simulink subsystem "FOC_Sub_CoreAlgoithm"  (R2025b)
settings: Solver=VariableStepAuto  StartTime=0.0  StopTime=10.0  RelTol=1e-3
PreLoadFcn:
  | FOC_Config;
undefined symbols (not defined in the file): innerPI, motor, outerPI, Tctr
libraries: mcbeeMathTransformLib x3, slpidlib x3, mcbcontrolslib x3, mcbpositiondecoderlib x2
settings Model: Creator=k  LastModifiedBy=k
settings SolverCC: AlgebraicLoopSolver=TrustRegion
settings DebuggingCC: UnconnectedInputMsg=warning  UnconnectedOutputMsg=warning  UnconnectedLineMsg=warning
settings ModelReferenceCC: EnableRefExpFcnMdlSchedulingChecks=on
settings RTWCC: GPUComputeCapability=3.5  DLArmComputeVersion=19.05

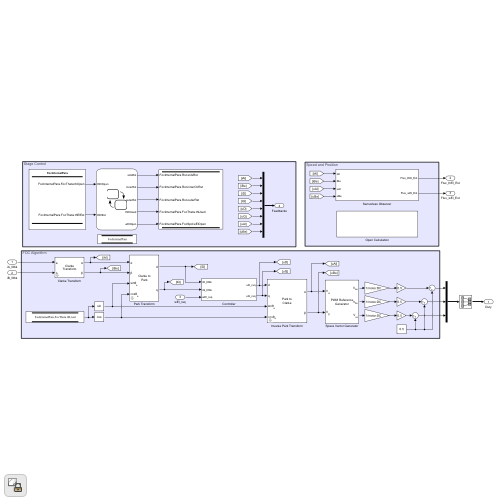
[thumbnail: Simulink's stored preview of the top-level diagram]
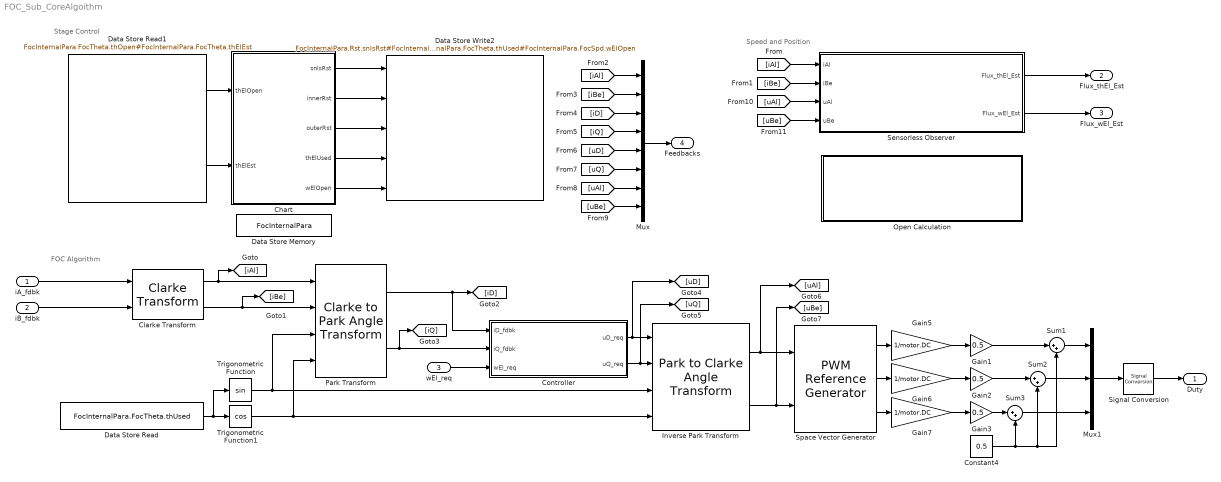
== system FOC_Sub_CoreAlgoithm ==
  note: Speed and Position
  note: Stage Control
  note: FOC Algorithm
  iA_fdbk : Inport
  iB_fdbk : Inport  Port=2
  wEl_req : Inport  Port=3
  Chart : Stateflow chart  TreatAsAtomicUnit=on
  Clarke Transform : mcbeeMathTransformLib/Clarke Transform  VariantControl=Variant2  PowerInvariant=off  UseWithEmbedded=on  PhaseInput=Two inputs
  Constant4 : Constant  Value=0.5  OutDataTypeStr=single
  Controller : Subsystem
  Data Store Memory : DataStoreMemory  DataStoreName=FocInternalPara  ReadBeforeWriteMsg=warning  WriteAfterWriteMsg=warning  WriteAfterReadMsg=warning  ShowAdditionalParam=off  OutDataTypeStr=Bus: strcutFocInternalPara
  Data Store Read : DataStoreRead  DataStoreName=FocInternalPara  DataStoreElements=FocInternalPara.FocTheta.thUsed  IndexOptions=Index vector (dialog)  Indices=1  OutputSizes=1
  Data Store Read1 : DataStoreRead  DataStoreName=FocInternalPara  DataStoreElements=FocInternalPara.FocTheta.thOpen#FocInternalPara.FocTheta.thElEst  IndexOptions=Index vector (dialog)  Indices=1  OutputSizes=1
  Data Store Write2 : DataStoreWrite  DataStoreName=FocInternalPara  DataStoreElements=FocInternalPara.Rst.snlsRst#FocInternalPara.Rst.innerCtrRst#FocInternalPara.Rst.outerRst#FocInternalPara.FocTheta.thUsed#FocInternalPara.FocSpd.wElOpen  IndexOptions=Index vector (dialog)  Indices=1  OutputSizes=1
  Gain1 : Gain  Gain=0.5  OutDataTypeStr=single
  Gain2 : Gain  Gain=0.5  OutDataTypeStr=single
  Gain3 : Gain  Gain=0.5  OutDataTypeStr=single
  Gain5 : Gain  Gain=1/motor.DC
  Gain6 : Gain  Gain=1/motor.DC
  Gain7 : Gain  Gain=1/motor.DC
  Inverse Park Transform : mcbeeMathTransformLib/Park to Clarke Angle Transform  AxisAlignment=D-axis  UseWithEmbedded=on  PhaseInput=Two inputs  ThetaInput=Sine and Cosine electrical position  AngleInput=Per-unit  N_points=1024
  Mux : Mux  Inputs=8
  Mux1 : Mux  Inputs=3
  Open Calculation : Subsystem
  Park Transform : mcbeeMathTransformLib/Clarke to Park Angle Transform  AxisAlignment=D-axis  UseWithEmbedded=on  PhaseInput=Two inputs  ThetaInput=Sine and Cosine electrical position  AngleInput=Per-unit  N_points=1024
  Sensorless Observer : Subsystem
  Signal Conversion : SignalConversion  OverrideOpt=off
  Space Vector Generator : mcbcontrolslib/PWM Reference Generator  inSignal=Valphabeta  modType=SVM: space vector modulation
  Sum1 : Sum  Inputs=|++
  Sum2 : Sum  Inputs=|++
  Sum3 : Sum  Inputs=|++
  Trigonometric Function : Trigonometry
  Trigonometric Function1 : Trigonometry  Operator=cos
  Duty : Outport  PortDimensions=3
  Flux_thEl_Est : Outport  Port=2
  Flux_wEl_Est : Outport  Port=3
  Feedbacks : Outport  Port=4
  wires:
  Signal Conversion/1 -> Duty/1
  Mux1/1 -> Signal Conversion/1
  Sum1/1 -> Mux1/1
  Sum3/1 -> Mux1/3
  Sum2/1 -> Mux1/2
  iB_fdbk/1 -> Clarke Transform/2
  iA_fdbk/1 -> Clarke Transform/1
  Clarke Transform/1 -> Park Transform/1, [iAl]
  Clarke Transform/2 -> [iBe], Park Transform/2
  Gain7/1 -> Gain3/1
  Constant4/1 -> Sum3/2, Sum2/2, Sum1/2
  Space Vector Generator/1 -> Gain5/1
  Space Vector Generator/2 -> Gain6/1
  Gain5/1 -> Gain1/1
  Gain1/1 -> Sum1/1
  Space Vector Generator/3 -> Gain7/1
  Gain2/1 -> Sum2/1
  Gain3/1 -> Sum3/1
  Gain6/1 -> Gain2/1
  Inverse Park Transform/1 -> Space Vector Generator/1, [uAl]
  Inverse Park Transform/2 -> [uBe], Space Vector Generator/2
  Sensorless Observer/1(Flux_thEl_Est) -> Flux_thEl_Est/1
  Sensorless Observer/2(Flux_wEl_Est) -> Flux_wEl_Est/1
  Park Transform/1 -> Controller/1(iD_fdbk), [iD]
  Park Transform/2 -> [iQ], Controller/2(iQ_fdbk)
  Controller/1(uD_req) -> Inverse Park Transform/1, [uD]
  Controller/2(uQ_req) -> [uQ], Inverse Park Transform/2
  Trigonometric Function1/1 -> Park Transform/4, Inverse Park Transform/4
  Data Store Read/1 -> Trigonometric Function/1, Trigonometric Function1/1
  Trigonometric Function/1 -> Park Transform/3, Inverse Park Transform/3
  wEl_req/1 -> Controller/3(wEl_req)
  Chart/3(outerRst) -> Data Store Write2/3
  Chart/2(innerRst) -> Data Store Write2/2
  Chart/1(snlsRst) -> Data Store Write2/1
  Data Store Read1/1 -> Chart/1(thElOpen)
  Data Store Read1/2 -> Chart/2(thElEst)
  Chart/4(thElUsed) -> Data Store Write2/4
  Chart/5(wElOpen) -> Data Store Write2/5
  [iAl] -> Sensorless Observer/1(iAl)
  [iBe] -> Sensorless Observer/2(iBe)
  [uAl] -> Sensorless Observer/3(uAl)
  [uBe] -> Sensorless Observer/4(uBe)
  [uBe] -> Mux/8
  [uAl] -> Mux/7
  [uQ] -> Mux/6
  [uD] -> Mux/5
  [iQ] -> Mux/4
  [iD] -> Mux/3
  [iBe] -> Mux/2
  [iAl] -> Mux/1
  Mux/1 -> Feedbacks/1

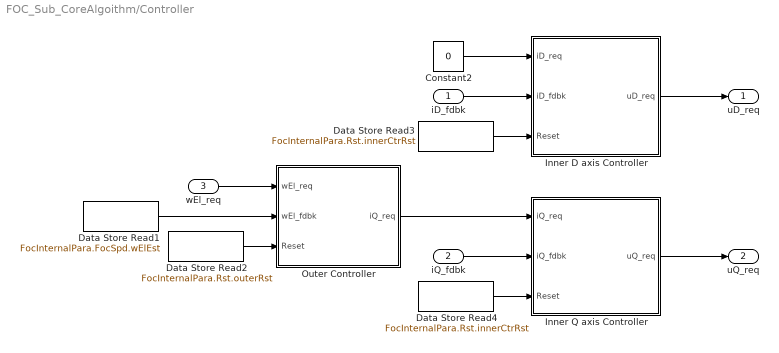
== system FOC_Sub_CoreAlgoithm/Controller ==
  iD_fdbk : Inport
  iQ_fdbk : Inport  Port=2
  wEl_req : Inport  Port=3
  Constant2 : Constant  Value=0  OutDataTypeStr=single
  Data Store Read1 : DataStoreRead  DataStoreName=FocInternalPara  DataStoreElements=FocInternalPara.FocSpd.wElEst  IndexOptions=Index vector (dialog)  Indices=1  OutputSizes=1
  Data Store Read2 : DataStoreRead  DataStoreName=FocInternalPara  DataStoreElements=FocInternalPara.Rst.outerRst  IndexOptions=Index vector (dialog)  Indices=1  OutputSizes=1
  Data Store Read3 : DataStoreRead  DataStoreName=FocInternalPara  DataStoreElements=FocInternalPara.Rst.innerCtrRst  IndexOptions=Index vector (dialog)  Indices=1  OutputSizes=1
  Data Store Read4 : DataStoreRead  DataStoreName=FocInternalPara  DataStoreElements=FocInternalPara.Rst.innerCtrRst  IndexOptions=Index vector (dialog)  Indices=1  OutputSizes=1
  Inner D axis Controller : Subsystem
  Inner Q axis Controller : Subsystem
  Outer Controller : Subsystem
  uD_req : Outport
  uQ_req : Outport  Port=2
  wires:
  Inner D axis Controller/1(uD_req) -> uD_req/1
  iD_fdbk/1 -> Inner D axis Controller/2(iD_fdbk)
  wEl_req/1 -> Outer Controller/1(wEl_req)
  Data Store Read1/1 -> Outer Controller/2(wEl_fdbk)
  Constant2/1 -> Inner D axis Controller/1(iD_req)
  Inner Q axis Controller/1(uQ_req) -> uQ_req/1
  Data Store Read2/1 -> Outer Controller/3(Reset)
  Outer Controller/1(iQ_req) -> Inner Q axis Controller/1(iQ_req)
  iQ_fdbk/1 -> Inner Q axis Controller/2(iQ_fdbk)
  Data Store Read3/1 -> Inner D axis Controller/3(Reset)
  Data Store Read4/1 -> Inner Q axis Controller/3(Reset)

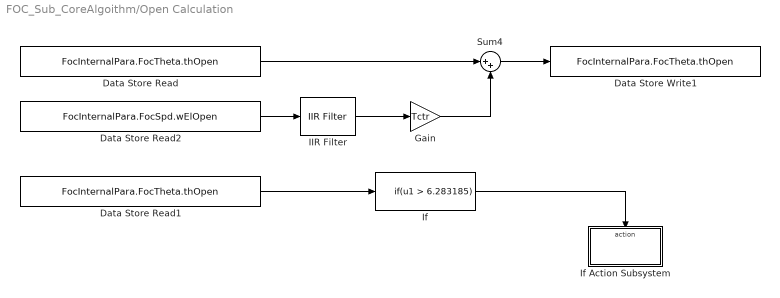
== system FOC_Sub_CoreAlgoithm/Open Calculation ==
  Data Store Read : DataStoreRead  DataStoreName=FocInternalPara  DataStoreElements=FocInternalPara.FocTheta.thOpen  IndexOptions=Index vector (dialog)  Indices=1  OutputSizes=1
  Data Store Read1 : DataStoreRead  DataStoreName=FocInternalPara  DataStoreElements=FocInternalPara.FocTheta.thOpen  IndexOptions=Index vector (dialog)  Indices=1  OutputSizes=1
  Data Store Read2 : DataStoreRead  DataStoreName=FocInternalPara  DataStoreElements=FocInternalPara.FocSpd.wElOpen  IndexOptions=Index vector (dialog)  Indices=1  OutputSizes=1
  Data Store Write1 : DataStoreWrite  DataStoreName=FocInternalPara  DataStoreElements=FocInternalPara.FocTheta.thOpen  IndexOptions=Index vector (dialog)  Indices=1  OutputSizes=1
  Gain : Gain  Gain=Tctr
  IIR Filter : mcbcontrolslib/IIR Filter  VariantControl=Low Pass Filter  VariantSelect=Low-pass  FilterConstantInputType=Specify via dialog  Filter_constant=0.002  InitialOutput=Specify via dialog  InitialOutputValue=0  ExternalReset=none  advancedSettings=off  Ts=50e-6  cutOff_freq=6.379
  If : If  IfExpression=u1 > 6.283185  ShowElse=off
  If Action Subsystem : Subsystem  TreatAsAtomicUnit=on
  Sum4 : Sum  Inputs=|++  OutDataTypeStr=single
  wires:
  If/1 -> If Action Subsystem/Action
  Data Store Read1/1 -> If/1
  Data Store Read/1 -> Sum4/1
  Sum4/1 -> Data Store Write1/1
  Data Store Read2/1 -> IIR Filter/1
  Gain/1 -> Sum4/2
  IIR Filter/1 -> Gain/1

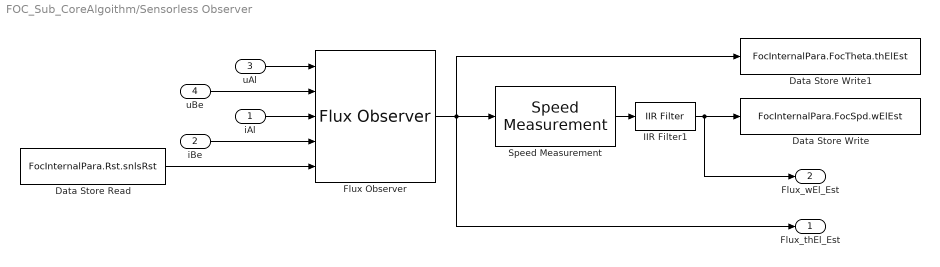
== system FOC_Sub_CoreAlgoithm/Sensorless Observer ==
  iAl : Inport
  iBe : Inport  Port=2
  uAl : Inport  Port=3
  uBe : Inport  Port=4
  Data Store Read : DataStoreRead  DataStoreName=FocInternalPara  DataStoreElements=FocInternalPara.Rst.snlsRst  IndexOptions=Index vector (dialog)  Indices=1  OutputSizes=1
  Data Store Write : DataStoreWrite  DataStoreName=FocInternalPara  DataStoreElements=FocInternalPara.FocSpd.wElEst  IndexOptions=Index vector (dialog)  Indices=1  OutputSizes=1
  Data Store Write1 : DataStoreWrite  DataStoreName=FocInternalPara  DataStoreElements=FocInternalPara.FocTheta.thElEst  IndexOptions=Index vector (dialog)  Indices=1  OutputSizes=1
  Flux Observer : mcbpositiondecoderlib/Flux Observer  DataTypeSelect=off  ParameterBusInput=off  MotorSelection=PMSM  BlockInputUnit=SI unit  PerUnitVoltage=13.86  PerUnitCurrent=19.3  PositionSelect=on  FluxSelect=off  TorqueSelect=off  PolePairs=4  StatorResistance=motor.Rs  StatorDAxisInductance=motor.L0*2  StatorLeakageInductance=0.0068  RotorLeakageInductance=0.0068  MagnetizingInductance=0.0300  CutoffFreq=3.1863  BlockSampleTime=Tctr  PositionUnit=Radians  PositionDatatype=single  FluxUnit=Weber  PerUnitFlux=0.1  FluxDatatype=single  TorqueUnit=Nm  PerUnitTorque=100  TorqueDatatype=single  DataType=0
  IIR Filter1 : mcbcontrolslib/IIR Filter  VariantControl=Low Pass Filter  VariantSelect=Low-pass  FilterConstantInputType=Specify via dialog  Filter_constant=0.001  InitialOutput=Specify via dialog  InitialOutputValue=0  ExternalReset=none  advancedSettings=off  Ts=50e-6  cutOff_freq=3.1863
  Speed Measurement : mcbpositiondecoderlib/Speed Measurement  DiscreteStepInput=off  LastDiscreteStepInput=off  PositionUnit=Radians  PositionScalingDatatype=uint32  SpeedCalculationMode=Time interval for speed calculation  TempSpeedCalculationMode=Time interval for speed calculation  SampleTimeAsync=Tctr  MaximumApplicationSpeed=1000  SpeedResolution=5e-6  DelayLength=20  MaximumMeasurableSpeed=22857.1429  MeasurableSpeedResolution=1.1176e-05  SpeedUnit=Radians/Sec  TempSpeedUnit=RPM  PerUnitSpeed=1000  SpeedDataType=single
  Flux_thEl_Est : Outport
  Flux_wEl_Est : Outport  Port=2
  wires:
  iBe/1 -> Flux Observer/4
  uBe/1 -> Flux Observer/2
  IIR Filter1/1 -> Data Store Write/1, Flux_wEl_Est/1
  Speed Measurement/1 -> IIR Filter1/1
  uAl/1 -> Flux Observer/1
  iAl/1 -> Flux Observer/3
  Data Store Read/1 -> Flux Observer/5
  Flux Observer/1 -> Speed Measurement/1, Flux_thEl_Est/1, Data Store Write1/1

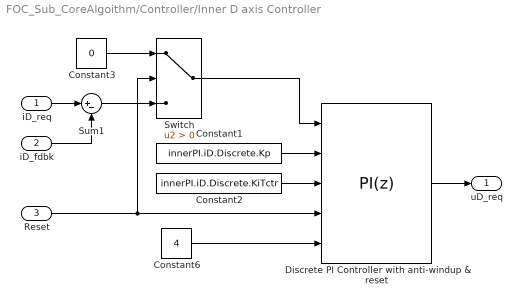
== system FOC_Sub_CoreAlgoithm/Controller/Inner D axis Controller ==
  iD_req : Inport
  iD_fdbk : Inport  Port=2
  Reset : Inport  Port=3
  Constant1 : Constant  Value=innerPI.iD.Discrete.Kp  OutDataTypeStr=single
  Constant2 : Constant  Value=innerPI.iD.Discrete.KiTctr  OutDataTypeStr=single
  Constant3 : Constant  Value=0  OutDataTypeStr=single
  Constant6 : Constant  Value=4  OutDataTypeStr=single
  Discrete PI Controller with anti-windup & reset : slpidlib/PID Controller  Controller=PI  Form=Parallel  TimeDomain=Discrete-time  UseExternalTs=off  SampleTime=-1  IntegratorMethod=Forward Euler  FilterMethod=Forward Euler  ControllerParametersSource=external  P=1  I=1  UseKiTs=on  D=0  UseExternalDerivativeSource=off  N=100  UseFilter=on  TunerSelectOption=Transfer Function Based (PID Tuner App)  InitialConditionSource=external  InitialConditionForIntegrator=0  InitialConditionForFilter=0  DifferentiatorICPrevScaledInput=0  ExternalReset=level  TrackingMode=off  Kt=1  LimitOutput=on  SatLimitsSource=internal  UpperSaturationLimit=10  LowerSaturationLimit=-10  LinearizeAsGain=on  AntiWindupMode=clamping  Kb=1  LimitIntegrator=off  UpperIntegratorSaturationLimit=inf  LowerIntegratorSaturationLimit=-inf  RndMeth=Simplest  POutMin=[]  POutMax=[]  IOutMin=[]  IOutMax=[]  DOutMin=[]  DOutMax=[]  NOutMin=[]  NOutMax=[]  SumOutMin=[]  SumOutMax=[]  SaturationOutDataTypeStr=Inherit: Inherit via back propagation  SaturationOutMin=[]  SaturationOutMax=[]  PParamMin=[]  PParamMax=[]  IParamMin=[]  IParamMax=[]  DParamMin=[]  DParamMax=[]  NParamMin=[]  NParamMax=[]  KbParamMin=[]  KbParamMax=[]  KtParamMin=[]  KtParamMax=[]  KbOutMin=[]  KbOutMax=[]  KtOutMin=[]  KtOutMax=[]  IntegratorOutMin=[]  IntegratorOutMax=[]  FilterOutMin=[]  FilterOutMax=[]  SumI1OutMin=[]  SumI1OutMax=[]  SumI2OutMin=[]  SumI2OutMax=[]  SumI3OutMin=[]  SumI3OutMax=[]  SumI4OutMin=[]  SumI4OutMax=[]  SumDOutMin=[]  SumDOutMax=[]  DifferentiatorOutMin=[]  DifferentiatorOutMax=[]  FilterDiffOutCoefMin=[]  FilterDiffOutCoefMax=[]  ReciprocalOutMin=[]  ReciprocalOutMax=[]  SumDenOutMin=[]  SumDenOutMax=[]  SumNumOutMin=[]  SumNumOutMax=[]  DivideOutMin=[]  DivideOutMax=[]  UdiffTsProdOutMin=[]  UdiffTsProdOutMax=[]  NTsProdOutMin=[]  NTsProdOutMax=[]  UintegralTsProdOutMin=[]  UintegralTsProdOutMax=[]  UngainTsProdOutMin=[]  UngainTsProdOutMax=[]  ClampingZeroOutDataTypeStr=Inherit: Inherit via back propagation  ClampingZeroOutMin=[]  ClampingZeroOutMax=[]  FilterDenConstantOutDataTypeStr=Inherit: Inherit via back propagation  FilterDenConstantOutMin=[]  FilterDenConstantOutMax=[]  PCopyOutDataTypeStr=Inherit: Inherit via back propagation  PCopyOutMin=[]  PCopyOutMax=[]  NCopyOutDataTypeStr=Inherit: Inherit via back propagation  NCopyOutMin=[]  NCopyOutMax=[]  IntegratorContinuousStateAttributes=''  IntegratorStateMustResolveToSignalObject=off  IntegratorRTWStateStorageClass=Auto  FilterContinuousStateAttributes=''  FilterStateMustResolveToSignalObject=off  FilterRTWStateStorageClass=Auto  ParallelPVariant=ExternalParameters  IdealPVariant=Disabled  IVariant=ExternalParameters  DVariant=Disabled  IntegratorVariant=Discrete  SatVariant=Enabled  AWVariant=DiscClampingParallel  PCopyVariant=Disabled  TRVariant=Disabled  FdbkBlocksVariant=Forward  IdealPFdbkVariant=Disabled  SatFdbkVariant=Disabled  DerivativeFilterVariant=Disabled  NVariant=Disabled  NCopyVariant=Disabled_SignalSpec  FilterICVariant=Disabled  IntegratorICVariant=ExternalICs  ExternalResetVariant=ExternalReset  TRSumVariant=Passthrough  SumFdbkVariant=Disabled  SumVariant=Sum_PI  TsampFilterVariant=InternalTs  TsampNgainVariant=Passthrough  TsampIntegralVariant=Disabled_SignalSpec  ExternalSaturationOutDataTypeStr=Inherit: Same as second input  DerivativeSourceVariant=Disabled  PreIntVariant=InternalPreInt
  Sum1 : Sum  Inputs=|+-
  Switch : Switch  Criteria=u2 > Threshold  SaturateOnIntegerOverflow=off  InputSameDT=off
  uD_req : Outport
  wires:
  Constant6/1 -> Discrete PI Controller with anti-windup & reset/5
  Discrete PI Controller with anti-windup & reset/1 -> uD_req/1
  Constant2/1 -> Discrete PI Controller with anti-windup & reset/3
  Constant1/1 -> Discrete PI Controller with anti-windup & reset/2
  Reset/1 -> Switch/2, Discrete PI Controller with anti-windup & reset/4
  Constant3/1 -> Switch/1
  iD_fdbk/1 -> Sum1/2
  Sum1/1 -> Switch/3
  iD_req/1 -> Sum1/1
  Switch/1 -> Discrete PI Controller with anti-windup & reset/1

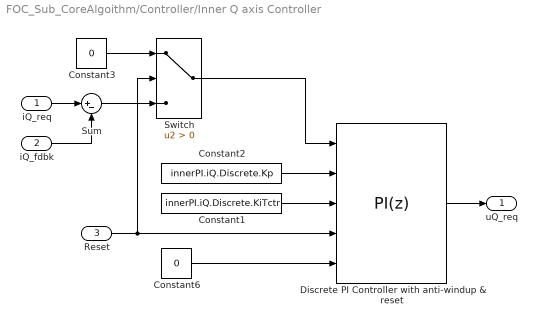
== system FOC_Sub_CoreAlgoithm/Controller/Inner Q axis Controller ==
  iQ_req : Inport
  iQ_fdbk : Inport  Port=2
  Reset : Inport  Port=3
  Constant1 : Constant  Value=innerPI.iQ.Discrete.KiTctr  OutDataTypeStr=single
  Constant2 : Constant  Value=innerPI.iQ.Discrete.Kp  OutDataTypeStr=single
  Constant3 : Constant  Value=0  OutDataTypeStr=single
  Constant6 : Constant  Value=0  OutDataTypeStr=single
  Discrete PI Controller with anti-windup & reset : slpidlib/PID Controller  Controller=PI  Form=Parallel  TimeDomain=Discrete-time  UseExternalTs=off  SampleTime=-1  IntegratorMethod=Forward Euler  FilterMethod=Forward Euler  ControllerParametersSource=external  P=1  I=1  UseKiTs=on  D=0  UseExternalDerivativeSource=off  N=100  UseFilter=on  TunerSelectOption=Transfer Function Based (PID Tuner App)  InitialConditionSource=external  InitialConditionForIntegrator=0  InitialConditionForFilter=0  DifferentiatorICPrevScaledInput=0  ExternalReset=level  TrackingMode=off  Kt=1  LimitOutput=on  SatLimitsSource=internal  UpperSaturationLimit=10  LowerSaturationLimit=-10  LinearizeAsGain=on  AntiWindupMode=clamping  Kb=1  LimitIntegrator=off  UpperIntegratorSaturationLimit=inf  LowerIntegratorSaturationLimit=-inf  RndMeth=Simplest  POutMin=[]  POutMax=[]  IOutMin=[]  IOutMax=[]  DOutMin=[]  DOutMax=[]  NOutMin=[]  NOutMax=[]  SumOutMin=[]  SumOutMax=[]  SaturationOutDataTypeStr=Inherit: Inherit via back propagation  SaturationOutMin=[]  SaturationOutMax=[]  PParamMin=[]  PParamMax=[]  IParamMin=[]  IParamMax=[]  DParamMin=[]  DParamMax=[]  NParamMin=[]  NParamMax=[]  KbParamMin=[]  KbParamMax=[]  KtParamMin=[]  KtParamMax=[]  KbOutMin=[]  KbOutMax=[]  KtOutMin=[]  KtOutMax=[]  IntegratorOutMin=[]  IntegratorOutMax=[]  FilterOutMin=[]  FilterOutMax=[]  SumI1OutMin=[]  SumI1OutMax=[]  SumI2OutMin=[]  SumI2OutMax=[]  SumI3OutMin=[]  SumI3OutMax=[]  SumI4OutMin=[]  SumI4OutMax=[]  SumDOutMin=[]  SumDOutMax=[]  DifferentiatorOutMin=[]  DifferentiatorOutMax=[]  FilterDiffOutCoefMin=[]  FilterDiffOutCoefMax=[]  ReciprocalOutMin=[]  ReciprocalOutMax=[]  SumDenOutMin=[]  SumDenOutMax=[]  SumNumOutMin=[]  SumNumOutMax=[]  DivideOutMin=[]  DivideOutMax=[]  UdiffTsProdOutMin=[]  UdiffTsProdOutMax=[]  NTsProdOutMin=[]  NTsProdOutMax=[]  UintegralTsProdOutMin=[]  UintegralTsProdOutMax=[]  UngainTsProdOutMin=[]  UngainTsProdOutMax=[]  ClampingZeroOutDataTypeStr=Inherit: Inherit via back propagation  ClampingZeroOutMin=[]  ClampingZeroOutMax=[]  FilterDenConstantOutDataTypeStr=Inherit: Inherit via back propagation  FilterDenConstantOutMin=[]  FilterDenConstantOutMax=[]  PCopyOutDataTypeStr=Inherit: Inherit via back propagation  PCopyOutMin=[]  PCopyOutMax=[]  NCopyOutDataTypeStr=Inherit: Inherit via back propagation  NCopyOutMin=[]  NCopyOutMax=[]  IntegratorContinuousStateAttributes=''  IntegratorStateMustResolveToSignalObject=off  IntegratorRTWStateStorageClass=Auto  FilterContinuousStateAttributes=''  FilterStateMustResolveToSignalObject=off  FilterRTWStateStorageClass=Auto  ParallelPVariant=ExternalParameters  IdealPVariant=Disabled  IVariant=ExternalParameters  DVariant=Disabled  IntegratorVariant=Discrete  SatVariant=Enabled  AWVariant=DiscClampingParallel  PCopyVariant=Disabled  TRVariant=Disabled  FdbkBlocksVariant=Forward  IdealPFdbkVariant=Disabled  SatFdbkVariant=Disabled  DerivativeFilterVariant=Disabled  NVariant=Disabled  NCopyVariant=Disabled_SignalSpec  FilterICVariant=Disabled  IntegratorICVariant=ExternalICs  ExternalResetVariant=ExternalReset  TRSumVariant=Passthrough  SumFdbkVariant=Disabled  SumVariant=Sum_PI  TsampFilterVariant=InternalTs  TsampNgainVariant=Passthrough  TsampIntegralVariant=Disabled_SignalSpec  ExternalSaturationOutDataTypeStr=Inherit: Same as second input  DerivativeSourceVariant=Disabled  PreIntVariant=InternalPreInt
  Sum : Sum  Inputs=|+-
  Switch : Switch  Criteria=u2 > Threshold  SaturateOnIntegerOverflow=off  InputSameDT=off
  uQ_req : Outport
  wires:
  iQ_fdbk/1 -> Sum/2
  iQ_req/1 -> Sum/1
  Constant2/1 -> Discrete PI Controller with anti-windup & reset/2
  Constant1/1 -> Discrete PI Controller with anti-windup & reset/3
  Sum/1 -> Switch/3
  Constant6/1 -> Discrete PI Controller with anti-windup & reset/5
  Reset/1 -> Switch/2, Discrete PI Controller with anti-windup & reset/4
  Discrete PI Controller with anti-windup & reset/1 -> uQ_req/1
  Constant3/1 -> Switch/1
  Switch/1 -> Discrete PI Controller with anti-windup & reset/1

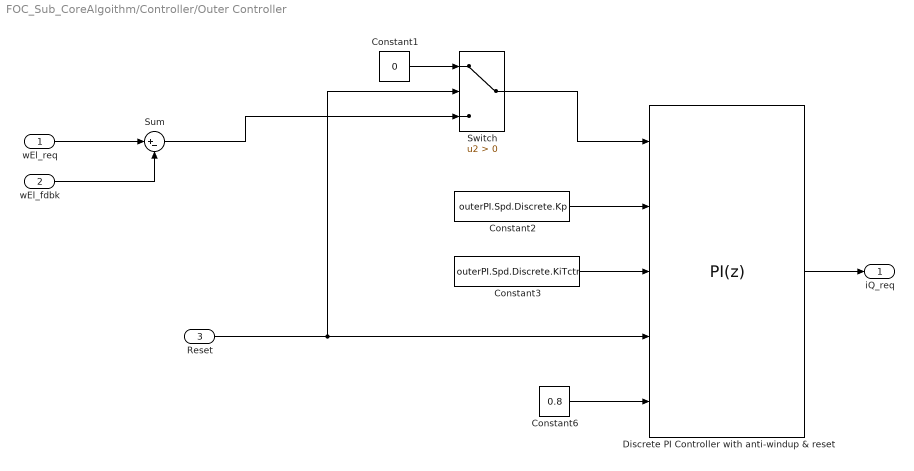
== system FOC_Sub_CoreAlgoithm/Controller/Outer Controller ==
  wEl_req : Inport
  wEl_fdbk : Inport  Port=2
  Reset : Inport  Port=3
  Constant1 : Constant  Value=0  OutDataTypeStr=single
  Constant2 : Constant  Value=outerPI.Spd.Discrete.Kp  OutDataTypeStr=single
  Constant3 : Constant  Value=outerPI.Spd.Discrete.KiTctr  OutDataTypeStr=single
  Constant6 : Constant  Value=0.8  OutDataTypeStr=single
  Discrete PI Controller with anti-windup & reset : slpidlib/PID Controller  Controller=PI  Form=Parallel  TimeDomain=Discrete-time  UseExternalTs=off  SampleTime=-1  IntegratorMethod=Forward Euler  FilterMethod=Forward Euler  ControllerParametersSource=external  P=1  I=1  UseKiTs=on  D=0  UseExternalDerivativeSource=off  N=100  UseFilter=on  TunerSelectOption=Transfer Function Based (PID Tuner App)  InitialConditionSource=external  InitialConditionForIntegrator=0  InitialConditionForFilter=0  DifferentiatorICPrevScaledInput=0  ExternalReset=level  TrackingMode=off  Kt=1  LimitOutput=on  SatLimitsSource=internal  UpperSaturationLimit=10  LowerSaturationLimit=-10  LinearizeAsGain=on  AntiWindupMode=clamping  Kb=1  LimitIntegrator=off  UpperIntegratorSaturationLimit=inf  LowerIntegratorSaturationLimit=-inf  RndMeth=Simplest  POutMin=[]  POutMax=[]  IOutMin=[]  IOutMax=[]  DOutMin=[]  DOutMax=[]  NOutMin=[]  NOutMax=[]  SumOutMin=[]  SumOutMax=[]  SaturationOutDataTypeStr=Inherit: Inherit via back propagation  SaturationOutMin=[]  SaturationOutMax=[]  PParamMin=[]  PParamMax=[]  IParamMin=[]  IParamMax=[]  DParamMin=[]  DParamMax=[]  NParamMin=[]  NParamMax=[]  KbParamMin=[]  KbParamMax=[]  KtParamMin=[]  KtParamMax=[]  KbOutMin=[]  KbOutMax=[]  KtOutMin=[]  KtOutMax=[]  IntegratorOutMin=[]  IntegratorOutMax=[]  FilterOutMin=[]  FilterOutMax=[]  SumI1OutMin=[]  SumI1OutMax=[]  SumI2OutMin=[]  SumI2OutMax=[]  SumI3OutMin=[]  SumI3OutMax=[]  SumI4OutMin=[]  SumI4OutMax=[]  SumDOutMin=[]  SumDOutMax=[]  DifferentiatorOutMin=[]  DifferentiatorOutMax=[]  FilterDiffOutCoefMin=[]  FilterDiffOutCoefMax=[]  ReciprocalOutMin=[]  ReciprocalOutMax=[]  SumDenOutMin=[]  SumDenOutMax=[]  SumNumOutMin=[]  SumNumOutMax=[]  DivideOutMin=[]  DivideOutMax=[]  UdiffTsProdOutMin=[]  UdiffTsProdOutMax=[]  NTsProdOutMin=[]  NTsProdOutMax=[]  UintegralTsProdOutMin=[]  UintegralTsProdOutMax=[]  UngainTsProdOutMin=[]  UngainTsProdOutMax=[]  ClampingZeroOutDataTypeStr=Inherit: Inherit via back propagation  ClampingZeroOutMin=[]  ClampingZeroOutMax=[]  FilterDenConstantOutDataTypeStr=Inherit: Inherit via back propagation  FilterDenConstantOutMin=[]  FilterDenConstantOutMax=[]  PCopyOutDataTypeStr=Inherit: Inherit via back propagation  PCopyOutMin=[]  PCopyOutMax=[]  NCopyOutDataTypeStr=Inherit: Inherit via back propagation  NCopyOutMin=[]  NCopyOutMax=[]  IntegratorContinuousStateAttributes=''  IntegratorStateMustResolveToSignalObject=off  IntegratorRTWStateStorageClass=Auto  FilterContinuousStateAttributes=''  FilterStateMustResolveToSignalObject=off  FilterRTWStateStorageClass=Auto  ParallelPVariant=ExternalParameters  IdealPVariant=Disabled  IVariant=ExternalParameters  DVariant=Disabled  IntegratorVariant=Discrete  SatVariant=Enabled  AWVariant=DiscClampingParallel  PCopyVariant=Disabled  TRVariant=Disabled  FdbkBlocksVariant=Forward  IdealPFdbkVariant=Disabled  SatFdbkVariant=Disabled  DerivativeFilterVariant=Disabled  NVariant=Disabled  NCopyVariant=Disabled_SignalSpec  FilterICVariant=Disabled  IntegratorICVariant=ExternalICs  ExternalResetVariant=ExternalReset  TRSumVariant=Passthrough  SumFdbkVariant=Disabled  SumVariant=Sum_PI  TsampFilterVariant=InternalTs  TsampNgainVariant=Passthrough  TsampIntegralVariant=Disabled_SignalSpec  ExternalSaturationOutDataTypeStr=Inherit: Same as second input  DerivativeSourceVariant=Disabled  PreIntVariant=InternalPreInt
  Sum : Sum  Inputs=|+-
  Switch : Switch  Criteria=u2 > Threshold  SaturateOnIntegerOverflow=off  InputSameDT=off
  iQ_req : Outport
  wires:
  Switch/1 -> Discrete PI Controller with anti-windup & reset/1
  Constant1/1 -> Switch/1
  Reset/1 -> Discrete PI Controller with anti-windup & reset/4, Switch/2
  Constant3/1 -> Discrete PI Controller with anti-windup & reset/3
  Constant2/1 -> Discrete PI Controller with anti-windup & reset/2
  Constant6/1 -> Discrete PI Controller with anti-windup & reset/5
  Sum/1 -> Switch/3
  wEl_req/1 -> Sum/1
  wEl_fdbk/1 -> Sum/2
  Discrete PI Controller with anti-windup & reset/1 -> iQ_req/1

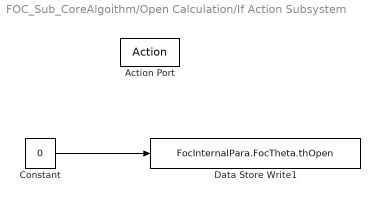
== system FOC_Sub_CoreAlgoithm/Open Calculation/If Action Subsystem ==
  Action Port : ActionPort
  Constant : Constant  Value=0  OutDataTypeStr=single
  Data Store Write1 : DataStoreWrite  DataStoreName=FocInternalPara  DataStoreElements=FocInternalPara.FocTheta.thOpen  IndexOptions=Index vector (dialog)  Indices=1  OutputSizes=1
  wires:
  Constant/1 -> Data Store Write1/1

== stateflow chart FOC_Sub_CoreAlgoithm/Chart ==
  state OpenStage
    outerRst = 1;
    snlsRst = 1;
    innerRst = 0;
    thElUsed = thElOpen;
    wElOpen = 94;
  state AlignStage
    outerRst = 1;
    snlsRst = 1;
    innerRst = 1;
    thElUsed = 0;
    wElOpen = 0;
  state RunStage
    outerRst = 0;
    snlsRst = 0;
    innerRst = 0;
    thElUsed = thElEst;
    wElOpen = 0;
  state TrackStage
    outerRst = 1;
    snlsRst = 0;
    innerRst = 0;
    thElUsed = thElOpen;
    wElOpen = 94;
  (default) -> AlignStage
  OpenStage -> TrackStage : after(8000, tick)
  AlignStage -> OpenStage : after(8000, tick)
  TrackStage -> RunStage : after(20000, tick)
  data: snlsRst output single; innerRst output single; outerRst output single; thElOpen input single; thElEst input single; thElUsed output single; wElOpen output single
